simulink model "Askhsh_12c"  (R2018b)
settings: Solver=VariableStepAuto  StartTime=0.0  StopTime=10  RelTol=1e-3
libraries: simulink x1
settings Model: Creator=Argy  LastModifiedBy=Argy
settings DataIOCC: Refine=10

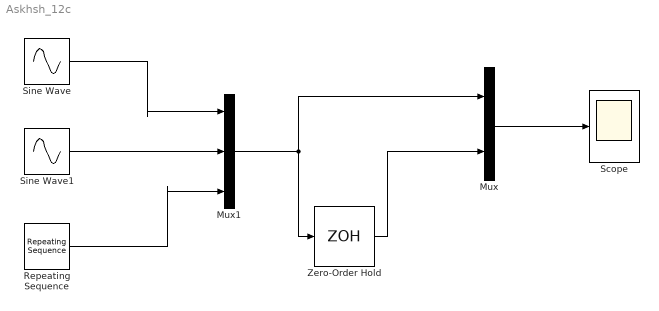
== system Askhsh_12c ==
  Mux : Mux  Inputs=2
  Mux1 : Mux  Inputs=3
  Repeating Sequence : simulink/Sources/Repeating Sequence  rep_seq_t=[0 2]  rep_seq_y=[0 -2]
  Scope : Scope
  Sine Wave : Sin  Amplitude=4  Frequency=10  SampleTime=0
  Sine Wave1 : Sin  Amplitude=2  Frequency=5  SampleTime=0
  Zero-Order Hold : ZeroOrderHold  SampleTime=0.1
  wires:
  Mux/1 -> Scope/1
  Zero-Order Hold/1 -> Mux/2
  Sine Wave/1 -> Mux1/1
  Sine Wave1/1 -> Mux1/2
  Mux1/1 -> Mux/1, Zero-Order Hold/1
  Repeating Sequence/1 -> Mux1/3
